simulink model "Duct_Bot_Motors"  (Simulink 7.3)
settings: Solver=FixedStepDiscrete  StartTime=0.0  StopTime=inf  FixedStep=1  RelTol=1e-3
undefined symbols (not defined in the file): S1, S2
settings Model: Creator=gclayton  LastModifiedBy=gclayton  SimulationMode=external
settings RTWCC: SystemTargetFile=rlnx.tlc  GenCodeOnly=on  TemplateMakefile=rlnx_ubuntu.tmf  Description=Linux Real-Time Target  ProcessScript=rlnx_make_rtw_hook
settings CodeAppCC: GenerateComments=off  SimulinkBlockComments=off
settings STFCustomTargetCC: ModelReferenceCompliant=off  MatFileLogging=on  SystemTargetFile=rlnx.tlc
settings GRTTargetCC: ModelReferenceCompliant=off  ParMdlRefBuildCompliant=off  CompOptLevelCompliant=off  ExtMode=on  ExtModeMexArgs='10.0.0.3'
settings CustomProperty: DataType=string  Value=/matlab_includes/libfreenect/build/lib/libfreenect.so -lm -ldl
settings EnumStrPairs: String=PC

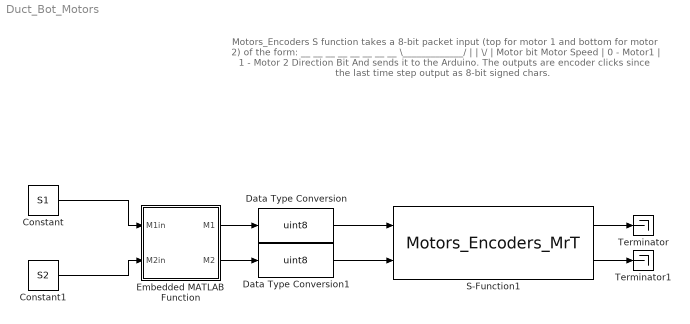
== system Duct_Bot_Motors ==
  note: Motors_Encoders S function takes a 8-bit packet input
      | (top for motor 1 and bottom for motor 2) of the form:
      |
      |          __ __ __ __ __ __ __ __
      |              \_____________/   |    |
      |                                \/                       |  Motor bit
      |                          Motor Speed             |   0 - Motor1
      |                                                             |   1 - Motor 2
      |                                      Direction Bit
      |
      | And sends it to the Arduino.  The outputs are encoder clicks
      | since the last time step output as 8-bit signed chars.
  Constant : Constant  Value=S1  OutDataType=fixdt(1, 16)  OutScaling=2^0
  Constant1 : Constant  Value=S2  OutDataType=fixdt(1, 16)  OutScaling=2^0
  Data Type Conversion : DataTypeConversion  OutDataTypeMode=uint8  OutDataType=fixdt(1, 16)  OutScaling=2^0  OutDataTypeStr=uint8
  Data Type Conversion1 : DataTypeConversion  OutDataTypeMode=uint8  OutDataType=fixdt(1, 16)  OutScaling=2^0  OutDataTypeStr=uint8
  Embedded MATLAB Function : Stateflow chart
  S-Function1 : S-Function  FunctionName=Motors_Encoders_MrT  EnableBusSupport=off
  Terminator : Terminator
  Terminator1 : Terminator
  wires:
  Embedded MATLAB Function/1(M1) -> Data Type Conversion/1
  Embedded MATLAB Function/2(M2) -> Data Type Conversion1/1
  Constant/1 -> Embedded MATLAB Function/1(M1in)
  Data Type Conversion/1 -> S-Function1/1
  Data Type Conversion1/1 -> S-Function1/2
  Constant1/1 -> Embedded MATLAB Function/2(M2in)
  S-Function1/1 -> Terminator/1
  S-Function1/2 -> Terminator1/1

== matlab function Embedded MATLAB Function ==
  data: M1in input double; M1 output double; M2in input double; M2 output double
function [M1, M2] = MotorPackets(M1in, M2in)
%#eml
if abs(M1in)>6
    M1in = sign(M1in)*6;
end

M1 = 0;
M2 = 1;

if M1in <= 0
    M1 = M1+2;
end

if M2in <= 0
    M2 = M2+2;
end
gain = 6/(2^6-1);
M1 = M1 + round(abs(M1in)/gain)*4;
M2 = M2 + round(abs(M2in)/gain)*4;
